simulink model "PaceMaker"  (R2022a)
settings: Solver=FixedStepAuto  StartTime=0.0  StopTime=inf  FixedStep=1e-3  RelTol=1e-3  EnableMultiTasking=on
undefined symbols (not defined in the file): D0, D1, D10, D11, D12, D13, D2, D3, D4, D5, D6, D7, D8, D9, PTA0, PTA1, PTA2, PTB23, PTB9, PTC16, PTC17, PTC2, PTC3, PTC4, PTD0, PTD1, PTD2, PTD3
libraries: frdmk64flib x14
settings Model: SimulationMode=external  ExtModeTrigDuration=5  Creator=22363  LastModifiedBy=22363
settings OptimizationCC: EnhancedBackFolding=on  PassReuseOutputArgsAs=Individual arguments  ZeroExternalMemoryAtStartup=off  ZeroInternalMemoryAtStartup=off  MaxStackSize=64  OptimizeBlockOrder=speed  DifferentSizesBufferReuse=on  OptimizationCustomize=off  EfficientTunableParamExpr=on
settings DebuggingCC: ParameterTunabilityLossMsg=error
settings HardwareCC: ProdBitPerPointer=32  ProdBitPerSizeT=32  ProdBitPerPtrDiffT=32  ProdLargestAtomicInteger=Long  ProdLargestAtomicFloat=Double  ProdWordSize=32  ProdHWDeviceType=ARM Compatible->ARM Cortex
settings SFSimCC: MATLABDynamicMemAlloc=off
settings RTWCC: SystemTargetFile=ert.tlc  HardwareBoard=NXP FRDM-K64F  TLCOptions="-aInlineSetEventsForThisBaseRateFcn=TLC_FALSE -aSuppressMultiTaskScheduler=TLC_FALSE  -aRateBasedStepFcn=0"  TemplateMakefile=ert_default_tmf  Toolchain=GNU Tools for ARM Embedded Processors
settings CodeAppCC: ForceParamTrailComments=on  IgnoreCustomStorageClasses=off  OperatorAnnotations=on  SimulinkDataObjDesc=on  SFDataObjDesc=on  InsertBlockDesc=on
settings ERTTargetCC: ExtModeTransport=6  ExtModeMexFile=sendToCommService

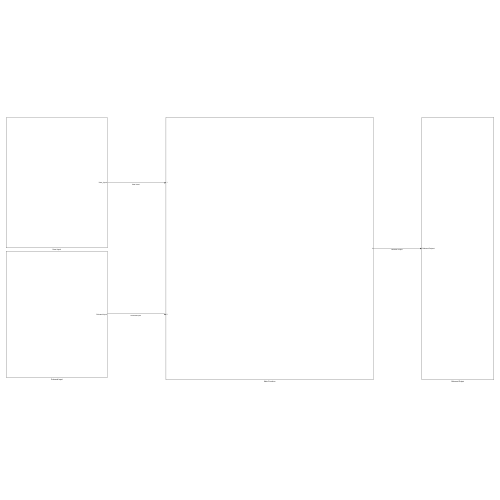
[thumbnail: Simulink's stored preview of the top-level diagram]
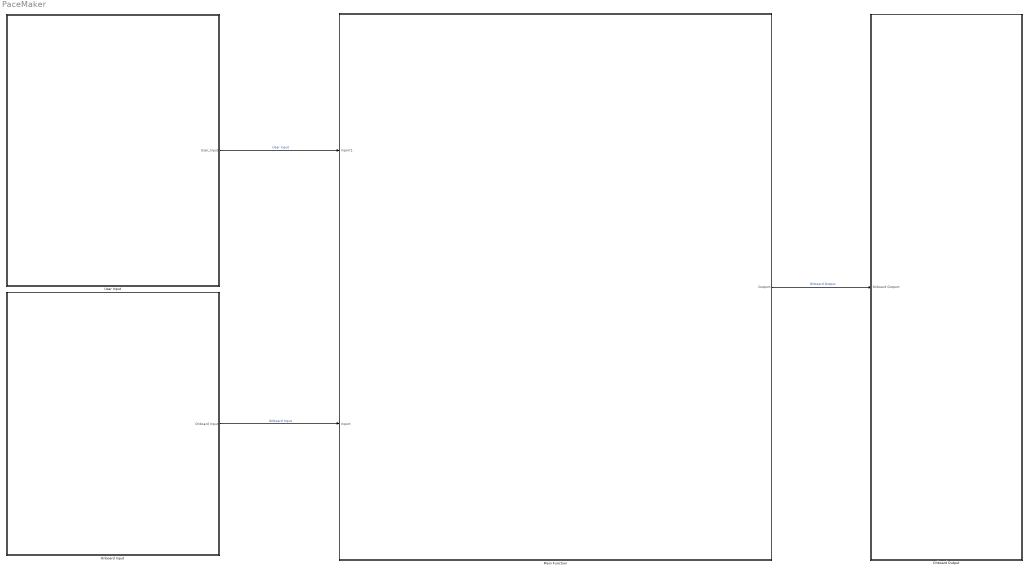
== system PaceMaker ==
  Main Function : Subsystem
  Onboard Input : Subsystem
  Onboard Output : Subsystem
  User Input : Subsystem
  wires:
  Main Function/1(Outport) -> Onboard Output/1(Onboard Outport)  "Onboard Output"
  User Input/1(User_Input) -> Main Function/1(Inport1)  "User Input"
  Onboard Input/1(Onboard Input) -> Main Function/2(Inport)  "Onboard Input"

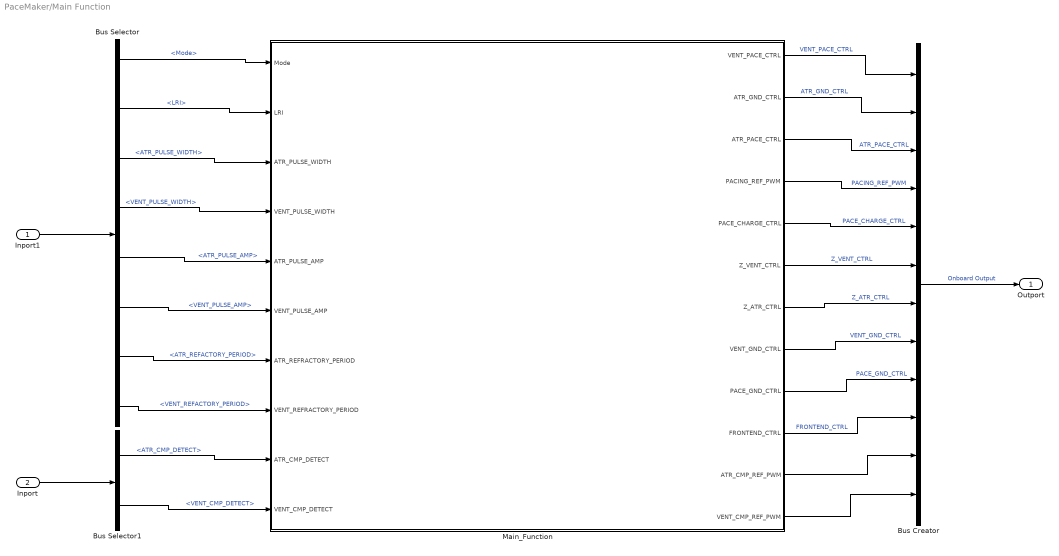
== system PaceMaker/Main Function ==
  Inport1 : Inport
  Inport : Inport  Port=2
  Bus Creator : BusCreator  Inputs=12
  Bus Selector : BusSelector  OutputSignals=Mode,LRI,ATR_PULSE_WIDTH,VENT_PULSE_WIDTH,ATR_PULSE_AMP,VENT_PULSE_AMP,ATR_REFACTORY_PERIOD,VENT_REFACTORY_PERIOD
  Bus Selector1 : BusSelector  OutputSignals=ATR_CMP_DETECT,VENT_CMP_DETECT
  Main_Function : Stateflow chart  TreatAsAtomicUnit=on
  Outport : Outport
  wires:
  Main_Function/8(VENT_GND_CTRL) -> Bus Creator/8  "VENT_GND_CTRL"
  Main_Function/1(VENT_PACE_CTRL) -> Bus Creator/1  "VENT_PACE_CTRL"
  Bus Selector/1 -> Main_Function/1(Mode)  "<Mode>"
  Bus Selector/2 -> Main_Function/2(LRI)  "<LRI>"
  Bus Selector/3 -> Main_Function/3(ATR_PULSE_WIDTH)  "<ATR_PULSE_WIDTH>"
  Bus Selector/4 -> Main_Function/4(VENT_PULSE_WIDTH)  "<VENT_PULSE_WIDTH>"
  Bus Selector1/1 -> Main_Function/9(ATR_CMP_DETECT)  "<ATR_CMP_DETECT>"
  Bus Selector1/2 -> Main_Function/10(VENT_CMP_DETECT)  "<VENT_CMP_DETECT>"
  Main_Function/9(PACE_GND_CTRL) -> Bus Creator/9  "PACE_GND_CTRL"
  Main_Function/7(Z_ATR_CTRL) -> Bus Creator/7  "Z_ATR_CTRL"
  Main_Function/6(Z_VENT_CTRL) -> Bus Creator/6  "Z_VENT_CTRL"
  Main_Function/5(PACE_CHARGE_CTRL) -> Bus Creator/5  "PACE_CHARGE_CTRL"
  Main_Function/4(PACING_REF_PWM) -> Bus Creator/4  "PACING_REF_PWM"
  Main_Function/3(ATR_PACE_CTRL) -> Bus Creator/3  "ATR_PACE_CTRL"
  Main_Function/2(ATR_GND_CTRL) -> Bus Creator/2  "ATR_GND_CTRL"
  Inport1/1 -> Bus Selector/1
  Inport/1 -> Bus Selector1/1
  Bus Creator/1 -> Outport/1  "Onboard Output"
  Bus Selector/7 -> Main_Function/7(ATR_REFRACTORY_PERIOD)  "<ATR_REFACTORY_PERIOD>"
  Bus Selector/8 -> Main_Function/8(VENT_REFRACTORY_PERIOD)  "<VENT_REFACTORY_PERIOD>"
  Bus Selector/5 -> Main_Function/5(ATR_PULSE_AMP)  "<ATR_PULSE_AMP>"
  Bus Selector/6 -> Main_Function/6(VENT_PULSE_AMP)  "<VENT_PULSE_AMP>"
  Main_Function/10(FRONTEND_CTRL) -> Bus Creator/10  "FRONTEND_CTRL"
  Main_Function/11(ATR_CMP_REF_PWM) -> Bus Creator/11
  Main_Function/12(VENT_CMP_REF_PWM) -> Bus Creator/12

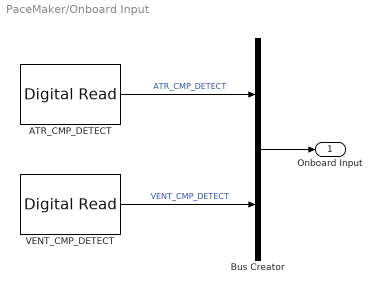
== system PaceMaker/Onboard Input ==
  ATR_CMP_DETECT : frdmk64flib/Digital Read  Whichpin=PTC16 (D0)  SampleTime=-1
  Bus Creator : BusCreator  Inputs=2
  VENT_CMP_DETECT : frdmk64flib/Digital Read  Whichpin=PTC17 (D1)  SampleTime=-1
  Onboard Input : Outport
  wires:
  VENT_CMP_DETECT/1 -> Bus Creator/2  "VENT_CMP_DETECT"
  ATR_CMP_DETECT/1 -> Bus Creator/1  "ATR_CMP_DETECT"
  Bus Creator/1 -> Onboard Input/1

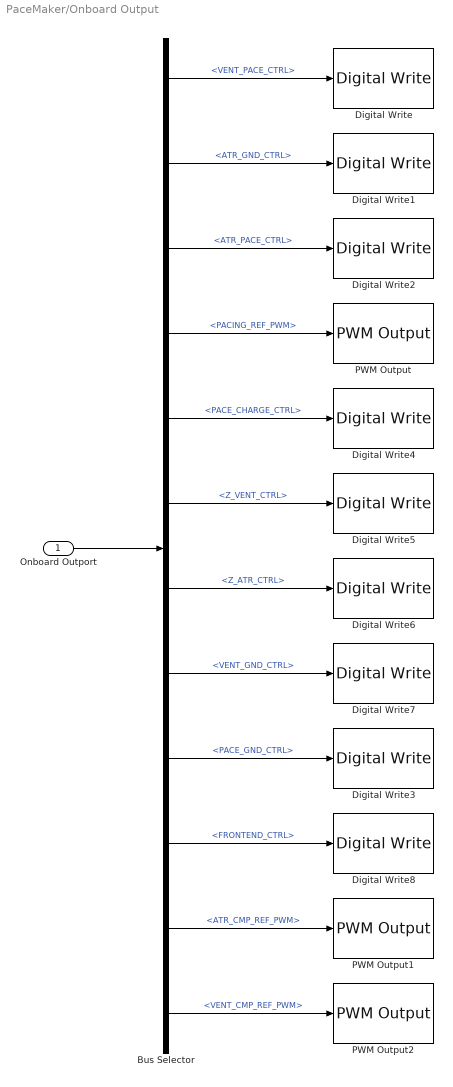
== system PaceMaker/Onboard Output ==
  Onboard Outport : Inport
  Bus Selector : BusSelector  OutputSignals=VENT_PACE_CTRL,ATR_GND_CTRL,ATR_PACE_CTRL,PACING_REF_PWM,PACE_CHARGE_CTRL,Z_VENT_CTRL,Z_ATR_CTRL,VENT_GND_CTRL,PACE_GND_CTRL,FRONTEND_CTRL,ATR_CMP_REF_PWM,VENT_CMP_REF_PWM
  Digital Write : frdmk64flib/Digital Write  Whichpin=PTC4 (D9)
  Digital Write1 : frdmk64flib/Digital Write  Whichpin=PTD2 (D11)
  Digital Write2 : frdmk64flib/Digital Write  Whichpin=PTA0 (D8)
  Digital Write3 : frdmk64flib/Digital Write  Whichpin=PTD0 (D10)
  Digital Write4 : frdmk64flib/Digital Write  Whichpin=PTB9 (D2)
  Digital Write5 : frdmk64flib/Digital Write  Whichpin=PTC3 (D7)
  Digital Write6 : frdmk64flib/Digital Write  Whichpin=PTB23 (D4)
  Digital Write7 : frdmk64flib/Digital Write  Whichpin=PTD3 (D12)
  Digital Write8 : frdmk64flib/Digital Write  Whichpin=PTD1 (D13)
  PWM Output : frdmk64flib/PWM Output  Whichpin=PTA2 (D5)  InitialFrequency=2000  InitialDutyCycle=50
  PWM Output1 : frdmk64flib/PWM Output  Whichpin=PTC2 (D6)  InitialFrequency=2000  InitialDutyCycle=50
  PWM Output2 : frdmk64flib/PWM Output  Whichpin=PTA1 (D3)  InitialFrequency=2000  InitialDutyCycle=50
  wires:
  Onboard Outport/1 -> Bus Selector/1
  Bus Selector/1 -> Digital Write/1  "<VENT_PACE_CTRL>"
  Bus Selector/2 -> Digital Write1/1  "<ATR_GND_CTRL>"
  Bus Selector/3 -> Digital Write2/1  "<ATR_PACE_CTRL>"
  Bus Selector/4 -> PWM Output/1  "<PACING_REF_PWM>"
  Bus Selector/5 -> Digital Write4/1  "<PACE_CHARGE_CTRL>"
  Bus Selector/6 -> Digital Write5/1  "<Z_VENT_CTRL>"
  Bus Selector/7 -> Digital Write6/1  "<Z_ATR_CTRL>"
  Bus Selector/8 -> Digital Write7/1  "<VENT_GND_CTRL>"
  Bus Selector/9 -> Digital Write3/1  "<PACE_GND_CTRL>"
  Bus Selector/10 -> Digital Write8/1  "<FRONTEND_CTRL>"
  Bus Selector/11 -> PWM Output1/1  "<ATR_CMP_REF_PWM>"
  Bus Selector/12 -> PWM Output2/1  "<VENT_CMP_REF_PWM>"

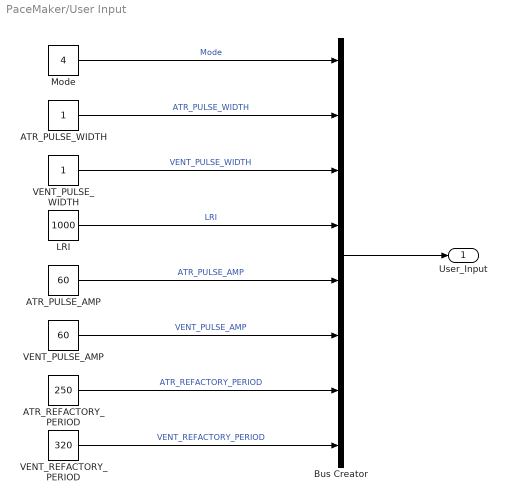
== system PaceMaker/User Input ==
  ATR_PULSE_AMP : Constant  Value=60
  ATR_PULSE_WIDTH : Constant
  ATR_REFACTORY_PERIOD : Constant  Value=250
  Bus Creator : BusCreator  Inputs=8
  LRI : Constant  Value=1000
  Mode : Constant  Value=4
  VENT_PULSE_AMP : Constant  Value=60
  VENT_PULSE_WIDTH : Constant
  VENT_REFACTORY_PERIOD : Constant  Value=320
  User_Input : Outport
  wires:
  LRI/1 -> Bus Creator/4  "LRI"
  VENT_PULSE_WIDTH/1 -> Bus Creator/3  "VENT_PULSE_WIDTH"
  ATR_PULSE_WIDTH/1 -> Bus Creator/2  "ATR_PULSE_WIDTH"
  Mode/1 -> Bus Creator/1  "Mode"
  ATR_REFACTORY_PERIOD/1 -> Bus Creator/7  "ATR_REFACTORY_PERIOD"
  VENT_REFACTORY_PERIOD/1 -> Bus Creator/8  "VENT_REFACTORY_PERIOD"
  Bus Creator/1 -> User_Input/1
  ATR_PULSE_AMP/1 -> Bus Creator/5  "ATR_PULSE_AMP"
  VENT_PULSE_AMP/1 -> Bus Creator/6  "VENT_PULSE_AMP"

== stateflow chart PaceMaker/Main Function/Main_Function ==
  state AAI_Mode
    entry:
    ATR_PACE_CTRL = 0;
    ATR_GND_CTRL = 1;
    %
    VENT_PACE_CTRL = 0;
    VENT_GND_CTRL = 0;
    %
    PACING_REF_PWM = ATR_PULSE_AMP;
    ATR_CMP_REF_PWM =80;
    PACE_CHARGE_CTRL = 1;
    %
    Z_VENT_CTRL = 0;
    Z_ATR_CTRL = 0;
    %
    FRONTEND_CTRL = 1;
    state SendPulse
      entry:
      PACE_CHARGE_CTRL = 0;
      PACE_GND_CTRL = 1;
      ATR_PACE_CTRL = 1;
      ATR_GND_CTRL = 0;
      VENT_PACE_CTRL = 0;
      VENT_GND_CTRL = 0;
      FRONTEND_CTRL = 0;
    state ReadyPulse
      entry:
      PACE_CHARGE_CTRL = 1;
      PACE_GND_CTRL = 1;
      ATR_PACE_CTRL = 0;
      ATR_GND_CTRL = 1;
      VENT_PACE_CTRL = 0;
      VENT_GND_CTRL = 0;
      FRONTEND_CTRL = 1;
    state Monitor_Pulse
      entry:
      PACE_CHARGE_CTRL = 1;
      PACE_GND_CTRL = 1;
      ATR_PACE_CTRL = 0;
      ATR_GND_CTRL = 1;
      VENT_PACE_CTRL = 0;
      VENT_GND_CTRL = 0;
      FRONTEND_CTRL = 1;
    (default) -> AAI_Mode.ReadyPulse
    AAI_Mode.SendPulse -> AAI_Mode.ReadyPulse : after(ATR_PULSE_WIDTH,msec)
    AAI_Mode.Monitor_Pulse -> AAI_Mode.ReadyPulse [order 2] : [ATR_CMP_DETECT == true]
    AAI_Mode.Monitor_Pulse -> AAI_Mode.SendPulse [order 1] : after(LRI-ATR_REFRACTORY_PERIOD-ATR_PULSE_WIDTH,msec)
    AAI_Mode.ReadyPulse -> AAI_Mode.Monitor_Pulse : after(ATR_REFRACTORY_PERIOD,msec)
  state AOO_Mode
    entry:
    ATR_PACE_CTRL = 0;
    ATR_GND_CTRL = 1;
    %
    VENT_PACE_CTRL = 0;
    VENT_GND_CTRL = 0;
    %
    PACING_REF_PWM = ATR_PULSE_AMP;
    PACE_CHARGE_CTRL = 1;
    %
    Z_VENT_CTRL = 0;
    Z_ATR_CTRL = 0;
    state ReadyPulse
      entry:
      PACE_CHARGE_CTRL = 1;
      PACE_GND_CTRL = 1;
      ATR_PACE_CTRL = 0;
      ATR_GND_CTRL = 1;
      VENT_PACE_CTRL = 0;
      VENT_GND_CTRL = 0;
    state SendPulse
      entry:
      PACE_CHARGE_CTRL = 0;
      PACE_GND_CTRL = 1;
      ATR_PACE_CTRL = 1;
      ATR_GND_CTRL = 0;
      VENT_PACE_CTRL = 0;
      VENT_GND_CTRL = 0;
    (default) -> AOO_Mode.ReadyPulse
    AOO_Mode.ReadyPulse -> AOO_Mode.SendPulse : after(LRI - ATR_PULSE_WIDTH,msec)
    AOO_Mode.SendPulse -> AOO_Mode.ReadyPulse : after(ATR_PULSE_WIDTH,msec)
  state Mode_Selector
    entry:
    ATR_PACE_CTRL = 0;
    ATR_GND_CTRL = 0;
    %
    VENT_PACE_CTRL = 0;
    VENT_GND_CTRL = 0;
    %
    PACE_CHARGE_CTRL = 0;
    PACE_CHARGE_CTRL = 0;
    %
    Z_VENT_CTRL = 0;
    Z_ATR_CTRL = 0;
    %
    FRONTEND_CTRL = 0;
  state AAI_Mode1
    entry:
    VENT_PACE_CTRL = 0;
    VENT_GND_CTRL = 1;
    %
    ATR_PACE_CTRL = 0;
    ATR_GND_CTRL = 0;
    %
    PACING_REF_PWM = VENT_PULSE_AMP;
    VENT_CMP_REF_PWM =80;
    PACE_CHARGE_CTRL = 1;
    %
    Z_VENT_CTRL = 0;
    Z_ATR_CTRL = 0;
    %
    FRONTEND_CTRL = 1;
    state SendPulse
      entry:
      PACE_CHARGE_CTRL = 0;
      PACE_GND_CTRL = 1;
      VENT_PACE_CTRL = 1;
      VENT_GND_CTRL = 0;
      ATR_PACE_CTRL = 0;
      ATR_GND_CTRL = 0;
      FRONTEND_CTRL = 0;
    state ReadyPulse
      entry:
      PACE_CHARGE_CTRL = 1;
      PACE_GND_CTRL = 1;
      VENT_PACE_CTRL = 0;
      VENT_GND_CTRL = 1;
      ATR_PACE_CTRL = 0;
      ATR_GND_CTRL = 0;
      FRONTEND_CTRL = 1;
    state Monitor_Pulse
      entry:
      PACE_CHARGE_CTRL = 1;
      PACE_GND_CTRL = 1;
      VENT_PACE_CTRL = 0;
      VENT_GND_CTRL = 1;
      ATR_PACE_CTRL = 0;
      ATR_GND_CTRL = 0;
      FRONTEND_CTRL = 1;
    (default) -> AAI_Mode1.ReadyPulse
    AAI_Mode1.SendPulse -> AAI_Mode1.ReadyPulse : after(VENT_PULSE_WIDTH,msec)
    AAI_Mode1.Monitor_Pulse -> AAI_Mode1.ReadyPulse [order 2] : [VENT_CMP_DETECT == true]
    AAI_Mode1.Monitor_Pulse -> AAI_Mode1.SendPulse [order 1] : after(LRI - VENT_REFRACTORY_PERIOD - VENT_PULSE_WIDTH,msec)
    AAI_Mode1.ReadyPulse -> AAI_Mode1.Monitor_Pulse : after(VENT_REFRACTORY_PERIOD,msec)
  state VOO_Mode
    entry:
    ATR_PACE_CTRL = 0;
    ATR_GND_CTRL = 0;
    %
    VENT_PACE_CTRL = 0;
    VENT_GND_CTRL = 1;
    %
    PACING_REF_PWM = VENT_PULSE_AMP;
    PACE_CHARGE_CTRL = 1;
    %
    Z_VENT_CTRL = 0;
    Z_ATR_CTRL = 0;
    state ReadyPulse
      entry:
      PACE_CHARGE_CTRL = 1;
      PACE_GND_CTRL = 1;
      ATR_PACE_CTRL = 0;
      ATR_GND_CTRL = 0;
      VENT_PACE_CTRL = 0;
      VENT_GND_CTRL = 1;
    state SendPulse
      entry:
      PACE_CHARGE_CTRL = 0;
      PACE_GND_CTRL = 1;
      ATR_PACE_CTRL = 0;
      ATR_GND_CTRL = 0;
      VENT_PACE_CTRL = 1;
      VENT_GND_CTRL = 0;
    (default) -> VOO_Mode.ReadyPulse
    VOO_Mode.SendPulse -> VOO_Mode.ReadyPulse : after(VENT_PULSE_WIDTH,msec)
    VOO_Mode.ReadyPulse -> VOO_Mode.SendPulse : after(LRI - VENT_PULSE_WIDTH,msec)
  Mode_Selector -> AAI_Mode [order 4] : [Mode == 3]
  Mode_Selector -> AOO_Mode [order 1] : [Mode == 1]
  (default) -> Mode_Selector
  Mode_Selector -> AAI_Mode1 [order 3] : [Mode == 4]
  Mode_Selector -> VOO_Mode [order 2] : [Mode == 2]
  data: VENT_PACE_CTRL output; ATR_GND_CTRL output; ATR_PACE_CTRL output; PACING_REF_PWM output; PACE_CHARGE_CTRL output; Z_VENT_CTRL output; Z_ATR_CTRL output; VENT_GND_CTRL output; Mode input; PACE_GND_CTRL output; LRI input double =1000; ATR_PULSE_WIDTH input double =0.4; VENT_PULSE_WIDTH input double =0.4; ATR_PULSE_AMP input; VENT_PULSE_AMP input; ATR_REFRACTORY_PERIOD input; VENT_REFRACTORY_PERIOD input; ATR_CMP_DETECT input; VENT_CMP_DETECT input; FRONTEND_CTRL output; ATR_CMP_REF_PWM output; VENT_CMP_REF_PWM output
